simulink library "vr_octavia_lib"  (Simulink 6.0)
settings: Solver=ode45  StartTime=0.0  StopTime=10.0  RelTol=1e-3
settings Model: Creator=Danek  LastModifiedBy=Danek
settings DataIOCC: SignalLoggingName=logsOut
settings DebuggingCC: CheckExecutionContextPreStartOutputMsg=on  CheckExecutionContextRuntimeOutputMsg=on
settings SFSimCC: SFSimApplyToAllLibs=on  SFSimBuildMode=Incremental

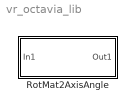
== system vr_octavia_lib ==
  RotMat2AxisAngle : Subsystem  PropExecContextAcrossSSBoundary=on
      mask Description:
      | Converts Rotation Matrix (defined columnwise as 9-element column vector) into
      | the Axis / Angle rotation representation used for defining rotations in VRML.
      mask Help:
      | Converts Rotation Matrix (defined columnwise as 9-element column vector) into
      | the Axis / Angle rotation representation used for defining rotations in VRML.
      mask Display:
      | text (0.1, 0.2, 'VR');
      | plot ([0.2 0.4 0.4 0.2 0.2], [0.4 0.4 0.8 0.8 0.4]);
      | plot ([0.25 0.25],[0.5 0.7]);
      | plot ([0.3 0.3],[0.5 0.7]);
      | plot ([0.35 0.35],[0.5 0.7]);
      | plot ([0.5 0.7 0.6 0.7 0.6], [0.6 0.6 0.7 0.6 0.5]);
      | plot ([0.8 0.9],[0.4 0.8]);

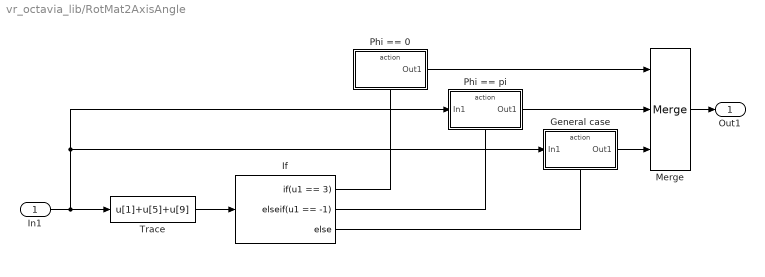
== system vr_octavia_lib/RotMat2AxisAngle ==
  In1 : Inport  LatchInput=off
  General case : Subsystem  TreatAsAtomicUnit=on  PropExecContextAcrossSSBoundary=on
  If : If  IfExpression=u1 == 3  ElseIfExpressions=u1 == -1
  Merge : Merge  Inputs=3
  Phi == 0 : Subsystem  TreatAsAtomicUnit=on  PropExecContextAcrossSSBoundary=on
  Phi == pi : Subsystem  TreatAsAtomicUnit=on  PropExecContextAcrossSSBoundary=on
  Trace : Fcn  Expr=u[1]+u[5]+u[9]
  Out1 : Outport
  wires:
  In1/1 -> General case/1(In1), Phi == pi/1(In1), Trace/1
  Trace/1 -> If/1
  If/1 -> Phi == 0/Action
  Phi == 0/1(Out1) -> Merge/1
  If/2 -> Phi == pi/Action
  If/3 -> General case/Action
  Phi == pi/1(Out1) -> Merge/2
  General case/1(Out1) -> Merge/3
  Merge/1 -> Out1/1

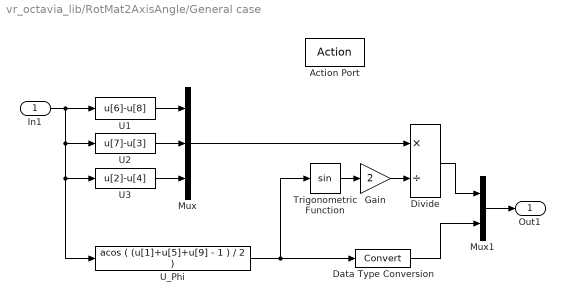
== system vr_octavia_lib/RotMat2AxisAngle/General case ==
  In1 : Inport  LatchInput=off
  Action Port : ActionPort
  Data Type Conversion : DataTypeConversion
  Divide : Product  Inputs=*/  OutScaling=2^-10
  Gain : Gain  Gain=2
  Mux : Mux  Inputs=3
  Mux1 : Mux  Inputs=2
  Trigonometric Function : Trigonometry
  U1 : Fcn  Expr=u[6]-u[8]
  U2 : Fcn  Expr=u[7]-u[3]
  U3 : Fcn  Expr=u[2]-u[4]
  U_Phi : Fcn  Expr=acos ( (u[1]+u[5]+u[9] - 1 ) / 2 )
  Out1 : Outport
  wires:
  Data Type Conversion/1 -> Mux1/2
  In1/1 -> U1/1, U2/1, U_Phi/1, U3/1
  Trigonometric Function/1 -> Gain/1
  U1/1 -> Mux/1
  U2/1 -> Mux/2
  U3/1 -> Mux/3
  Mux/1 -> Divide/1
  Gain/1 -> Divide/2
  Mux1/1 -> Out1/1
  Divide/1 -> Mux1/1
  U_Phi/1 -> Data Type Conversion/1, Trigonometric Function/1

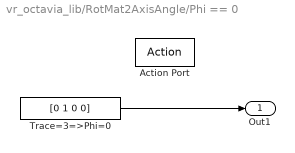
== system vr_octavia_lib/RotMat2AxisAngle/Phi == 0 ==
  Action Port : ActionPort
  Trace=3=>Phi=0 : Constant  Value=[0 1 0 0]  SampleTime=Inf
  Out1 : Outport  InitialOutput=[0 1 0 0]
  wires:
  Trace=3=>Phi=0/1 -> Out1/1

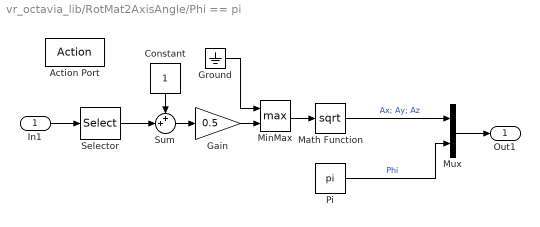
== system vr_octavia_lib/RotMat2AxisAngle/Phi == pi ==
  In1 : Inport  LatchInput=off
  Action Port : ActionPort
  Constant : Constant  Orientation=down
  Gain : Gain  Gain=0.5
  Ground : Ground
  Math Function : Math  Operator=sqrt  SaturateOnIntegerOverflow=on
  MinMax : MinMax  Function=max  Inputs=2
  Mux : Mux  Inputs=2
  Pi : Constant  Value=pi  SampleTime=Inf
  Selector : Selector  Elements=[1 5 9]  InputPortWidth=9
  Sum : Sum  Inputs=++|
  Out1 : Outport  InitialOutput=[0 0 0 pi]
  wires:
  Pi/1 -> Mux/2  "Phi"
  Sum/1 -> Gain/1
  Selector/1 -> Sum/2
  Constant/1 -> Sum/1
  In1/1 -> Selector/1
  Mux/1 -> Out1/1
  Ground/1 -> MinMax/1
  Gain/1 -> MinMax/2
  MinMax/1 -> Math Function/1
  Math Function/1 -> Mux/1  "Ax; Ay; Az"
